simulink model "Pruebas_filtrado"  (R2023a)
settings: Solver=VariableStepAuto  StartTime=0.0  StopTime=10.0  RelTol=1e-3
undefined symbols (not defined in the file): area_mem, c, k, m, perm, Q, r1, rho, v_sonido
libraries: dspvision x8, matrix_library x2
settings Model: Creator=tobip  LastModifiedBy=tobip

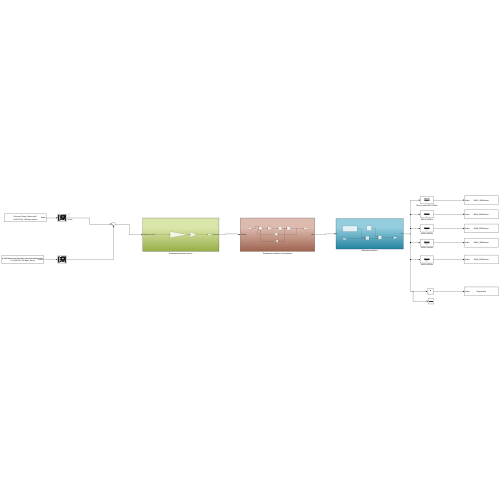
[thumbnail: Simulink's stored preview of the top-level diagram]
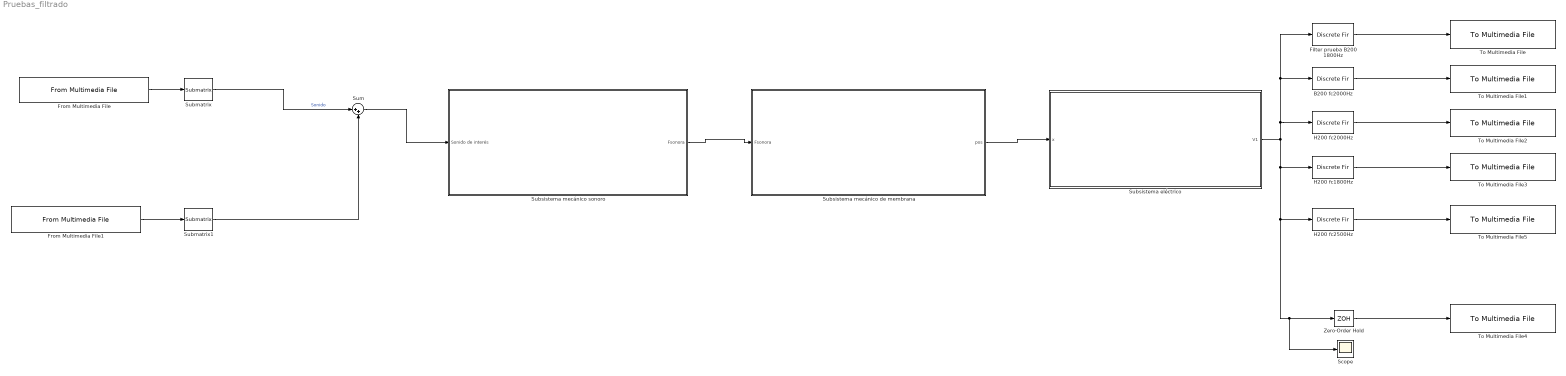
== system Pruebas_filtrado ==
  B200 fc2000Hz : DiscreteFir  Tag=BlockMethodSubSystem  Coefficients=[0 1.83057635375754512e-08 3.9529007824523685e-07 1.55910825338038789e-06 3.76770700347280875e-06 7.00736329359619744e-06 1.09301472211687974e-05 1.4844315408215566e-05 1.77655305137500905e-05 1.85292010987128519e-05 1.59558880344514605e-05 9.05351667491030031e-06 -2.7669734919763228e-06 -1.94909778736170261e-05 -4.03452156527393192e-05 -6.37177359122503275e-05 -8.71772893596150811e-05 -0.000107607705489954177 -0.000121461037604667137 -0.000125119129713206301 -0.00011533824121933605 -8.9737048689934339e-05 -4.72764906051115484e-05 1.13277343256887893e-05 8.33211540989788003e-05 0.000163811300849358454 0.000245897505370778666 0.000321054904994628207 0.000379773002469954496 0.000412420370303513424 0.000410277127099175438 0.000366648795812870806 0.000277952495146994354 0.000144652401776155501 -2.80811625062568753e-05 -0.00023010391289930311 -0.000446511161442282904 -0.00065838478644652382 -0.000844076565212307432 -0.000980974526958496712 -0.00104764052042331129 -0.0010261524961506232 -0.000904440360161047098 -0.000678375664469714869 -0.000353367905481524172 5.47627560112626412e-05 0.000519823673353936831 0.00100631867070531005 0.00147157958214806021 0.00186888998582014263 0.00215142314215150668 0.0022767133593484196 0.00221129290853706428 0.00193506566023672459 0.00144496277257264816 0.000757441428466622615 -9.05522644027214745e-05 -0.00104243167681747502 -0.00202476361787535565 -0.00295197284349670453 -0.00373273820378257045 -0.00427767907271705671 -0.00450776716828892639 -0.00436277149387703355 -0.00380896827277194547 -0.00284533525194545934 -0.00150750753258089903 0.000131098923597614361 0.00196139536568537597 0.00384411106834258321 0.00561853446011574206 0.00711407563955569148 0.0081639374286082908 0.00861993695209126859 0.00836733790251404513 0.00733845575045821187 0.00552379870738605762 0.00297961298967878768 -0.000169090212282736659 -0.00373064792249232615 -0.00745424786945846941 -0.0110426519744962343 -0.014169542947791134 -0.0165004897060302136 -0.0177161792309364872 -0.0175363045202477016 -0.0157423560813510256 -0.0121975549697943882 -0.00686229521671183774 0.00019627223707184758 0.00880149950810594182 0.0186718569629473648 0.0294328842772442548 0.0406359114198129104 0.0517824642469816923 0.0623528191737367302 0.071836827562594352 0.0797649223620647413 0.0857371659568155337 0.0894483057559149752 0.0907070664032905288 0.0894483057559149752 0.0857371659568155337 0.0797649223620647413 0.071836827562594352 0.0623528191737367302 0.0517824642469816923 0.0406359114198129104 0.0294328842772442548 0.0186718569629473648 0.00880149950810594182 0.00019627223707184758 -0.00686229521671183774 -0.0121975549697943882 -0.0157423560813510256 -0.0175363045202477016 -0.0177161792309364872 -0.0165004897060302136 -0.014169542947791134 -0.0110426519744962343 -0.00745424786945846941 -0.00373064792249232615 -0.000169090212282736659 0.00297961298967878768 0.00552379870738605762 0.00733845575045821187 0.00836733790251404513 0.00861993695209126859 0.0081639374286082908 0.00711407563955569148 0.00561853446011574206 0.00384411106834258321 0.00196139536568537597 0.000131098923597614361 -0.00150750753258089903 -0.00284533525194545934 -0.00380896827277194547 -0.00436277149387703355 -0.00450776716828892639 -0.00427767907271705671 -0.00373273820378257045 -0.00295197284349670453 -0.00202476361787535565 -0.00104243167681747502 -9.05522644027214745e-05 0.000757441428466622615 0.00144496277257264816 0.00193506566023672459 0.00221129290853706428 0.0022767133593484196 0.00215142314215150668 0.00186888998582014263 0.00147157958214806021 0.00100631867070531005 0.000519823673353936831 5.47627560112626412e-05 -0.000353367905481524172 -0.000678375664469714869 -0.000904440360161047098 -0.0010261524961506232 -0.00104764052042331129 -0.000980974526958496712 -0.000844076565212307432 -0.00065838478644652382 -0.000446511161442282904 -0.00023010391289930311 -2.80811625062568753e-05 0.000144652401776155501 0.000277952495146994354 0.000366648795812870806 ...(+728 chars)]
  Filter prueba B200 1800Hz : DiscreteFir  Tag=BlockMethodSubSystem  Coefficients=[0 7.24652832356188521e-08 -5.23782624738498232e-21 -6.675282150919552e-07 -2.32546562504132773e-06 -5.22190617674366559e-06 -9.37733204941596823e-06 -1.4527706576905175e-05 -2.01007077336600721e-05 -2.52320533236906118e-05 -2.88252060978315019e-05 -2.96534017283023188e-05 -2.6498240094570269e-05 -1.83144121829550524e-05 -4.40593566309191823e-06 1.54040110773000882e-05 4.06295112706107006e-05 7.00246916130837713e-05 0.000101551267711213309 0.000132425504936716578 0.000159253511256795893 0.0001782563263626227 0.000185577567562698827 0.000177657087576513136 0.000151644992748178274 0.000105822358223222479 3.99889794418797231e-05 -4.42246228702613387e-05 -0.000143163264147117697 -0.000251109024373292349 -0.000360428112608801501 -0.000461919012043696911 -0.000545362153558650252 -0.000600252917994597559 -0.000616680343502945365 -0.000586295162295064564 -0.00050329451282442371 -0.000365338677713132186 -0.000174309134435351917 6.31816048541805392e-05 0.000335608615422232262 0.000626744332221180946 0.000916296815277115062 0.00118098198325041642 0.00139599888422081014 0.00153683874273655131 0.00158132134999411258 0.00151171967909026245 0.00131680872185280088 0.000993660462994502055 0.000549006037692828888 -5.23858216267076414e-18 -0.000625749283419984518 -0.00129097558227676866 -0.00195041367344615476 -0.00255329274289711142 -0.00304656623940272649 -0.00337871086093326223 -0.00350386418207273816 -0.00338601897112400215 -0.0030029577118563691 -0.00234959755634923809 -0.00144042689350537285 -0.000310751257379701705 0.000983472150475005278 0.00236734806897806026 0.00375033978205100739 0.00503107008862271367 0.00610343054338352304 0.00686368997109162039 0.00721819371505886577 0.0070911673067812946 0.00643208958308969393 0.00522208638057725105 0.003478820226725245 0.0012594147242814646 -0.00133894744173130914 -0.00418098162670087811 -0.00709788532458695363 -0.00989444929475008506 -0.0123584203896081185 -0.0142716739206102325 -0.0154226072289702174 -0.0156190518302271718 -0.0147009285229756335 -0.0125518451123454357 -0.00910886369362379905 -0.00436974405197646659 0.00160290171592188872 0.00868093767594213007 0.0166737074043384961 0.0253346820739495972 0.0343714961426604612 0.0434588964341573319 0.0522539379494202996 0.0604126052508057593 0.0676069327234389422 0.0735416483032019369 0.0779693774867079442 0.0807035176445665414 0.0816280227514124129 0.0807035176445665414 0.0779693774867079442 0.0735416483032019369 0.0676069327234389422 0.0604126052508057593 0.0522539379494202996 0.0434588964341573319 0.0343714961426604612 0.0253346820739495972 0.0166737074043384961 0.00868093767594213007 0.00160290171592188872 -0.00436974405197646659 -0.00910886369362379905 -0.0125518451123454357 -0.0147009285229756335 -0.0156190518302271718 -0.0154226072289702174 -0.0142716739206102325 -0.0123584203896081185 -0.00989444929475008506 -0.00709788532458695363 -0.00418098162670087811 -0.00133894744173130914 0.0012594147242814646 0.003478820226725245 0.00522208638057725105 0.00643208958308969393 0.0070911673067812946 0.00721819371505886577 0.00686368997109162039 0.00610343054338352304 0.00503107008862271367 0.00375033978205100739 0.00236734806897806026 0.000983472150475005278 -0.000310751257379701705 -0.00144042689350537285 -0.00234959755634923809 -0.0030029577118563691 -0.00338601897112400215 -0.00350386418207273816 -0.00337871086093326223 -0.00304656623940272649 -0.00255329274289711142 -0.00195041367344615476 -0.00129097558227676866 -0.000625749283419984518 -5.23858216267076414e-18 0.000549006037692828888 0.000993660462994502055 0.00131680872185280088 0.00151171967909026245 0.00158132134999411258 0.00153683874273655131 0.00139599888422081014 0.00118098198325041642 0.000916296815277115062 0.000626744332221180946 0.000335608615422232262 6.31816048541805392e-05 -0.000174309134435351917 -0.000365338677713132186 -0.00050329451282442371 -0.000586295162295064564 -0.000616680343502945365 -0.000600252917994597559 -0.000545362153558650252 -0.000461919012043696911 ...(+733 chars)]
  From Multimedia File : dspvision/From Multimedia File  inputFilename=C:\Users\tobip\Documents\Control\Proyecto final\Audios dato\Discurso Roger Federer.mp3  readRange=[1 Inf]  loop=on  numPlays=1  outputStreams=Audio only  videoDataType=single  audioDataType=double  inheritSampleTime=on  userDefinedSampleTime=1/30  noAudioOutput=off  isIntensityVideo=off  fourcc=RGB  colorVideoFormat=Separate color signals  outputEOF=off  dataOrg=Column-major  audioFrameSize=1  computeAudioFrameSize=off  outSamplingMode=Sample based
      settings: LibrarySourceBlock=audiosources/From Multimedia File
  From Multimedia File1 : dspvision/From Multimedia File  inputFilename="C:\\Users\\tobip\\Downloads\\SOUND TEST  Royal Kludge S98 Mechanical Keyboard  #mechanicalkeyboard #asmr #keyboardasmr.mp3"  readRange=[1 Inf]  loop=on  numPlays=1  outputStreams=Audio only  videoDataType=single  audioDataType=double  inheritSampleTime=on  userDefinedSampleTime=1/30  noAudioOutput=off  isIntensityVideo=off  fourcc=RGB  colorVideoFormat=Separate color signals  outputEOF=off  dataOrg=Column-major  audioFrameSize=1  computeAudioFrameSize=off  outSamplingMode=Sample based
      settings: LibrarySourceBlock=audiosources/From Multimedia File
  H200 fc1800Hz : DiscreteFir  Tag=BlockMethodSubSystem  Coefficients=[0.000125144152077349865 6.55264979454243913e-05 -1.1928449595075705e-18 -6.83901465280600042e-05 -0.000136269006698061518 -0.000199973113165685608 -0.000255629840022287083 -0.000299287833587119601 -0.000327105580066830188 -0.000335597355428931708 -0.000321926737929569169 -0.000284228564314821627 -0.000221931780473618134 -0.000136049177898820524 -2.93965026581621075e-05 9.32963704991064338e-05 0.000225415156474266428 0.0003586561921956684 0.000483398865949644736 0.000589252190195314212 0.000665755112196383557 0.000703192663917076425 0.000693473870545317696 0.000631004152122332206 0.000513476331769485922 0.000342501599337603194 0.000124005748483605664 -0.000131672942477848446 -0.000410029933214454132 -0.000693006664109050655 -0.000959962440028376009 -0.00118896881882130448 -0.00135835854081060772 -0.00144843274272150402 -0.00144320705446259324 -0.00133206158162837832 -0.00111115370345444913 -0.000784457413035421418 -0.000364309158718417855 0.000128632509547874459 0.000666068975282595264 0.00121339582261732661 0.00173165014658894882 0.00217998070081169967 0.0025185022759167076 0.00271135389508317913 0.00272974895554655046 0.00255478756305092293 0.00217979941026834323 0.00161200099580237604 0.000873283895944795764 -8.17439618338273891e-18 -0.000958327393114875967 -0.00194136463977817521 -0.0028813205209989221 -0.00370713177714371766 -0.00434924972973165999 -0.00474473500174085999 -0.00484232267261183996 -0.00460709648053868846 -0.00402441097573624611 -0.00310272635241341755 -0.00187507182465818491 -0.000398927828788208565 0.00124558876449312825 0.0029592442394156958 0.00462880478626750708 0.00613352741007223198 0.00735269463181347643 0.00817377102749296952 0.00850069090071298161 0.00826174632438347184 0.00741653758906620202 0.00596147589663096993 0.00393339080958109068 0.00141089003132639302 -0.00148675819863240233 -0.00460330624474856055 -0.00775170191879439099 -0.0107225283839265835 -0.0132943289691928781 -0.0152453025580199207 -0.0163657475850653711 -0.0164705594208111074 -0.0154110528832169125 -0.0130853922150659333 -0.00944696582268950667 -0.00451014028254429974 0.0016470372712465548 0.00888345462203491039 0.0169989488099266221 0.0257416054434631905 0.0348180363283676492 0.043906149993609353 0.0526697761275188581 0.0607743863640084134 0.0679030780334831663 0.0737719596013683004 0.0781440988215156562 0.0808412662978824359 0.0817528242727317417 0.0808412662978824359 0.0781440988215156562 0.0737719596013683004 0.0679030780334831663 0.0607743863640084134 0.0526697761275188581 0.043906149993609353 0.0348180363283676492 0.0257416054434631905 0.0169989488099266221 0.00888345462203491039 0.0016470372712465548 -0.00451014028254429974 -0.00944696582268950667 -0.0130853922150659333 -0.0154110528832169125 -0.0164705594208111074 -0.0163657475850653711 -0.0152453025580199207 -0.0132943289691928781 -0.0107225283839265835 -0.00775170191879439099 -0.00460330624474856055 -0.00148675819863240233 0.00141089003132639302 0.00393339080958109068 0.00596147589663096993 0.00741653758906620202 0.00826174632438347184 0.00850069090071298161 0.00817377102749296952 0.00735269463181347643 0.00613352741007223198 0.00462880478626750708 0.0029592442394156958 0.00124558876449312825 -0.000398927828788208565 -0.00187507182465818491 -0.00310272635241341755 -0.00402441097573624611 -0.00460709648053868846 -0.00484232267261183996 -0.00474473500174085999 -0.00434924972973165999 -0.00370713177714371766 -0.0028813205209989221 -0.00194136463977817521 -0.000958327393114875967 -8.17439618338273891e-18 0.000873283895944795764 0.00161200099580237604 0.00217979941026834323 0.00255478756305092293 0.00272974895554655046 0.00271135389508317913 0.0025185022759167076 0.00217998070081169967 0.00173165014658894882 0.00121339582261732661 0.000666068975282595264 0.000128632509547874459 -0.000364309158718417855 -0.000784457413035421418 -0.00111115370345444913 -0.00133206158162837832 -0.00144320705446259324 -0.00144843274272150402 -0.00135835854081060772 -0.00118896881882130448 ...(+758 chars)]
  H200 fc2000Hz : DiscreteFir  Tag=BlockMethodSubSystem  Coefficients=[-5.56928887965323996e-05 1.65011438245537004e-05 8.97404129389855278e-05 0.000159235323802665862 0.00022009162972417537 0.000267507778546905491 0.000297028076662561244 0.00030485366062257119 0.000288200030555739591 0.000245675511305965986 0.000177641669329940406 8.6506699720296273e-05 -2.31018469780051173e-05 -0.00014433637834937926 -0.000268342086729793134 -0.000384707364236210015 -0.00048215215755155206 -0.000549426670478966937 -0.000576363543252263362 -0.000554999408859523633 -0.000480660081578202522 -0.000352890851136748013 -0.000176112058154881163 4.01080891230722538e-05 0.0002812463338075579 0.000528528322799664608 0.000760142225443803492 0.000952907949042803453 0.00108429460403765884 0.00113463045342545839 0.00108931159601457291 0.00094079311035012215 0.000690143237104743116 0.000347959694228160642 -6.55123016736293336e-05 -0.000521160190085571311 -0.000982705755809358409 -0.00140926525119598289 -0.00175861601479996091 -0.001990934889977244 -0.00207270564165747606 -0.00198044699745618087 -0.00170389625705465349 -0.00124829972377997456 -0.000635511796707235511 9.63124522686815125e-05 0.000894536087431914602 0.00169534580071897009 0.0024283810074139326 0.00302238837764083959 0.00341148451645994577 0.00354151851327269909 0.00337597368177574393 0.00290084170646281786 0.00212794664955293479 0.00109629064041346963 -0.000128867164522033134 -0.00145931071589772685 -0.00278945929549263881 -0.00400395802404863912 -0.00498677619654774081 -0.00563115432140427145 -0.00584961657959357211 -0.00558319945973669973 -0.00480904907338582793 -0.00354561337216146395 -0.00185479953038198927 0.000159326606607727535 0.00235546635562724864 0.00456352016844470149 0.00659611134894932602 0.00826250699229939302 0.00938400051612865889 0.00980963996366138874 0.00943108496947073389 0.0081953652910344444 0.00611440066924413047 0.00327032343009041803 -0.000184088132840851902 -0.00403022302427255476 -0.00799367568943868192 -0.0117590911319403208 -0.0149890162285861283 -0.0173456171069947714 -0.0185138545635019809 -0.0182245363907261523 -0.0162756038401307805 -0.0125500678039269838 -0.00702918815483403927 0.000200222721545358193 0.0089451122912353586 0.0189124119976689584 0.029721990975099373 0.0409256801261550299 0.052031266702432348 0.0625299886144426165 0.0719257851026266215 0.079764407724826486 0.0856604757140051049 0.0893206756611368557 0.0905615500562179931 0.0893206756611368557 0.0856604757140051049 0.079764407724826486 0.0719257851026266215 0.0625299886144426165 0.052031266702432348 0.0409256801261550299 0.029721990975099373 0.0189124119976689584 0.0089451122912353586 0.000200222721545358193 -0.00702918815483403927 -0.0125500678039269838 -0.0162756038401307805 -0.0182245363907261523 -0.0185138545635019809 -0.0173456171069947714 -0.0149890162285861283 -0.0117590911319403208 -0.00799367568943868192 -0.00403022302427255476 -0.000184088132840851902 0.00327032343009041803 0.00611440066924413047 0.0081953652910344444 0.00943108496947073389 0.00980963996366138874 0.00938400051612865889 0.00826250699229939302 0.00659611134894932602 0.00456352016844470149 0.00235546635562724864 0.000159326606607727535 -0.00185479953038198927 -0.00354561337216146395 -0.00480904907338582793 -0.00558319945973669973 -0.00584961657959357211 -0.00563115432140427145 -0.00498677619654774081 -0.00400395802404863912 -0.00278945929549263881 -0.00145931071589772685 -0.000128867164522033134 0.00109629064041346963 0.00212794664955293479 0.00290084170646281786 0.00337597368177574393 0.00354151851327269909 0.00341148451645994577 0.00302238837764083959 0.0024283810074139326 0.00169534580071897009 0.000894536087431914602 9.63124522686815125e-05 -0.000635511796707235511 -0.00124829972377997456 -0.00170389625705465349 -0.00198044699745618087 -0.00207270564165747606 -0.001990934889977244 -0.00175861601479996091 -0.00140926525119598289 -0.000982705755809358409 -0.000521160190085571311 -6.55123016736293336e-05 0.000347959694228160642 0.000690143237104743116 0.00094079311035012215 ...(+746 chars)]
  H200 fc2500Hz : DiscreteFir  Tag=BlockMethodSubSystem  Coefficients=[-0.000222219654175347933 -0.00016713260248594442 -8.98386782436484487e-05 1.91697880446349961e-06 9.84938717358789783e-05 0.000189065394371969089 0.000262527463652970051 0.000308585790394740977 0.000318960639621033353 0.000288600843402469522 0.000216755433258305189 0.000107723331772103536 -2.89001256335634088e-05 -0.000178629125966477619 -0.000323227645559331889 -0.000442567896166785033 -0.000517073814759191593 -0.000530497797835864215 -0.000472679060991016374 -0.000341871552165944471 -0.000146225142841473909 9.59343406577812602e-05 0.000357252721145095314 0.000603966002838980946 0.000799816186097935524 0.000910869813197802847 0.000910654086539299163 0.000784898833532098831 0.000535137832794225056 0.000180496787282985482 -0.000242820635784740701 -0.000684557736527415797 -0.00108580598881455478 -0.00138628427142167528 -0.00153266661538948158 -0.00148688272659393598 -0.00123319980156176199 -0.000782939588635876552 -0.000175901173348981608 0.000522066685543438815 0.00122540827311379014 0.00183863298362061376 0.00226849554459951103 0.00243712074849465957 0.00229433153109552838 0.00182738143565141543 0.00106648268057752847 8.49547274292785834e-05 -0.00100654388567213019 -0.0020714670482251743 -0.00296347519384215601 -0.00354539645838435882 -0.00370872499658596441 -0.00339104456585172069 -0.00258881727862926613 -0.00136338342892156333 0.000161248065834023005 0.00180925121760636782 0.00337178072798474627 0.00463189257941077747 0.00539278916699099595 0.00550591104782995316 0.00489512654576100027 0.00357347560063950385 0.00164961414811859398 -0.000677774824423426681 -0.00313790286286872583 -0.00541684492576247761 -0.00719473081735844122 -0.00818704297118046792 -0.00818504486482293792 -0.0070900771606230038 -0.00493681982928594054 -0.0019016261105760544 0.00170639592290751959 0.00547190649426861683 0.00891566065535334337 0.0115487576548134342 0.0129331888571965949 0.0127418859968334366 0.0108110440795465348 0.00717790670795971381 0.00209845275346322085 -0.00395859288765791281 -0.0103424836566119449 -0.0162741893452420516 -0.0209186979262467009 -0.0234690771989587085 -0.0232338027481298511 -0.0197180570724383927 -0.0126899180454171472 -0.00222359600521813668 0.0112859584750549594 0.0271398857517130346 0.0443832262145853265 0.0618799305399147584 0.0784083036741115985 0.0927677904482030746 0.103886623127320873 0.110919569765483991 0.113325893127411592 0.110919569765483991 0.103886623127320873 0.0927677904482030746 0.0784083036741115985 0.0618799305399147584 0.0443832262145853265 0.0271398857517130346 0.0112859584750549594 -0.00222359600521813668 -0.0126899180454171472 -0.0197180570724383927 -0.0232338027481298511 -0.0234690771989587085 -0.0209186979262467009 -0.0162741893452420516 -0.0103424836566119449 -0.00395859288765791281 0.00209845275346322085 0.00717790670795971381 0.0108110440795465348 0.0127418859968334366 0.0129331888571965949 0.0115487576548134342 0.00891566065535334337 0.00547190649426861683 0.00170639592290751959 -0.0019016261105760544 -0.00493681982928594054 -0.0070900771606230038 -0.00818504486482293792 -0.00818704297118046792 -0.00719473081735844122 -0.00541684492576247761 -0.00313790286286872583 -0.000677774824423426681 0.00164961414811859398 0.00357347560063950385 0.00489512654576100027 0.00550591104782995316 0.00539278916699099595 0.00463189257941077747 0.00337178072798474627 0.00180925121760636782 0.000161248065834023005 -0.00136338342892156333 -0.00258881727862926613 -0.00339104456585172069 -0.00370872499658596441 -0.00354539645838435882 -0.00296347519384215601 -0.0020714670482251743 -0.00100654388567213019 8.49547274292785834e-05 0.00106648268057752847 0.00182738143565141543 0.00229433153109552838 0.00243712074849465957 0.00226849554459951103 0.00183863298362061376 0.00122540827311379014 0.000522066685543438815 -0.000175901173348981608 -0.000782939588635876552 -0.00123319980156176199 -0.00148688272659393598 -0.00153266661538948158 -0.00138628427142167528 -0.00108580598881455478 -0.000684557736527415797 ...(+756 chars)]
  Scope : Scope
  Submatrix : matrix_library/Submatrix  RowSpan=All rows  RowStartMode=First  RowStartIndex=1  RowEndMode=Middle  RowEndIndex=1  ColSpan=One column  ColStartMode=First  ColStartIndex=1  ColEndMode=Last  ColEndIndex=1
  Submatrix1 : matrix_library/Submatrix  RowSpan=All rows  RowStartMode=First  RowStartIndex=1  RowEndMode=Last  RowEndIndex=1  ColSpan=One column  ColStartMode=First  ColStartIndex=1  ColEndMode=Last  ColEndIndex=1
  Subsistema eléctrico : Subsystem
  Subsistema mecánico de membrana : Subsystem
  Subsistema mecánico sonoro : Subsystem
  Sum : Sum  Inputs=|++
  To Multimedia File : dspvision/To Multimedia File  outputFilename=B200_1800Hz.wav  streamSelection=Audio only  videoCompressor=None (uncompressed)  audioCompressor=None (uncompressed)  imagePorts=Separate color signals  fileType=WAV  audioDatatype=16-bit integer  fourcc=RGB  videoQuality=75  mj2000CompFactor=10
      settings: LibrarySourceBlock=audiosinks/To Multimedia File
  To Multimedia File1 : dspvision/To Multimedia File  outputFilename=B200_2000Hz.wav  streamSelection=Audio only  videoCompressor=None (uncompressed)  audioCompressor=None (uncompressed)  imagePorts=Separate color signals  fileType=WAV  audioDatatype=16-bit integer  fourcc=RGB  videoQuality=75  mj2000CompFactor=10
      settings: LibrarySourceBlock=audiosinks/To Multimedia File
  To Multimedia File2 : dspvision/To Multimedia File  outputFilename=H200_2000Hz.wav  streamSelection=Audio only  videoCompressor=None (uncompressed)  audioCompressor=None (uncompressed)  imagePorts=Separate color signals  fileType=WAV  audioDatatype=16-bit integer  fourcc=RGB  videoQuality=75  mj2000CompFactor=10
      settings: LibrarySourceBlock=audiosinks/To Multimedia File
  To Multimedia File3 : dspvision/To Multimedia File  outputFilename=H200_1800Hz.wav  streamSelection=Audio only  videoCompressor=None (uncompressed)  audioCompressor=None (uncompressed)  imagePorts=Separate color signals  fileType=WAV  audioDatatype=16-bit integer  fourcc=RGB  videoQuality=75  mj2000CompFactor=10
      settings: LibrarySourceBlock=audiosinks/To Multimedia File
  To Multimedia File4 : dspvision/To Multimedia File  outputFilename=Original.wav  streamSelection=Audio only  videoCompressor=None (uncompressed)  audioCompressor=None (uncompressed)  imagePorts=Separate color signals  fileType=WAV  audioDatatype=16-bit integer  fourcc=RGB  videoQuality=75  mj2000CompFactor=10
      settings: LibrarySourceBlock=audiosinks/To Multimedia File
  To Multimedia File5 : dspvision/To Multimedia File  outputFilename=H200_2500Hz.wav  streamSelection=Audio only  videoCompressor=None (uncompressed)  audioCompressor=None (uncompressed)  imagePorts=Separate color signals  fileType=WAV  audioDatatype=16-bit integer  fourcc=RGB  videoQuality=75  mj2000CompFactor=10
      settings: LibrarySourceBlock=audiosinks/To Multimedia File
  Zero-Order Hold : ZeroOrderHold  SampleTime=1/44100
  wires:
  Subsistema mecánico sonoro/1(Fsonora) -> Subsistema mecánico de membrana/1(Fsonora)
  Sum/1 -> Subsistema mecánico sonoro/1(Sonido de interés)
  Subsistema mecánico de membrana/1(pos) -> Subsistema eléctrico/1(x)
  Submatrix/1 -> Sum/1  "Sonido"
  Submatrix1/1 -> Sum/2
  From Multimedia File/1 -> Submatrix/1
  From Multimedia File1/1 -> Submatrix1/1
  Filter prueba B200 1800Hz/1 -> To Multimedia File/1
  Subsistema eléctrico/1(V1) -> Scope/1, Zero-Order Hold/1, H200 fc2500Hz/1, H200 fc1800Hz/1, H200 fc2000Hz/1, B200 fc2000Hz/1, Filter prueba B200 1800Hz/1
  H200 fc1800Hz/1 -> To Multimedia File3/1
  B200 fc2000Hz/1 -> To Multimedia File1/1
  H200 fc2000Hz/1 -> To Multimedia File2/1
  Zero-Order Hold/1 -> To Multimedia File4/1
  H200 fc2500Hz/1 -> To Multimedia File5/1

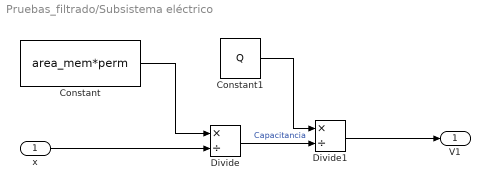
== system Pruebas_filtrado/Subsistema eléctrico ==
  x : Inport
  Constant : Constant  Value=area_mem*perm
  Constant1 : Constant  Value=Q
  Divide : Product  Inputs=*/
  Divide1 : Product  Inputs=*/
  V1 : Outport
  wires:
  x/1 -> Divide/2
  Constant/1 -> Divide/1
  Divide/1 -> Divide1/2  "Capacitancia"
  Divide1/1 -> V1/1
  Constant1/1 -> Divide1/1

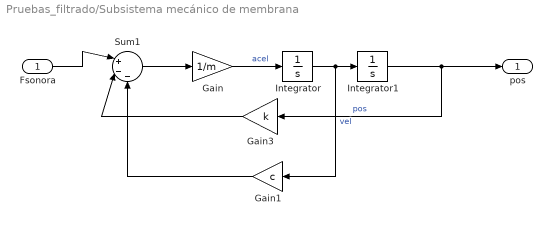
== system Pruebas_filtrado/Subsistema mecánico de membrana ==
  Fsonora : Inport
  Gain : Gain  Gain=1/m
  Gain1 : Gain  Gain=c
  Gain3 : Gain  Gain=k
  Integrator : Integrator
  Integrator1 : Integrator
  Sum1 : Sum  Inputs=|+--
  pos : Outport
  wires:
  Integrator1/1 -> Gain3/1, pos/1  "pos"
  Integrator/1 -> Gain1/1, Integrator1/1  "vel"
  Fsonora/1 -> Sum1/1
  Gain3/1 -> Sum1/2
  Sum1/1 -> Gain/1
  Gain/1 -> Integrator/1  "acel"
  Gain1/1 -> Sum1/3

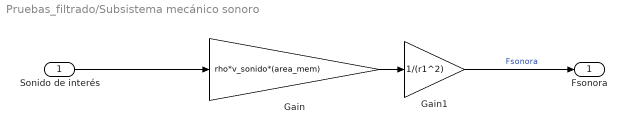
== system Pruebas_filtrado/Subsistema mecánico sonoro ==
  Sonido de interés : Inport
  Gain : Gain  Gain=rho*v_sonido*(area_mem)
  Gain1 : Gain  Gain=1/(r1^2)
  Fsonora : Outport
  wires:
  Gain/1 -> Gain1/1
  Sonido de interés/1 -> Gain/1
  Gain1/1 -> Fsonora/1  "Fsonora"
